simulink model "boostconv"  (R2024a)
settings: Solver=VariableStepAuto  StartTime=0.0  StopTime=10.0  RelTol=1e-3
undefined symbols (not defined in the file): c, l, r, vin
libraries: simulink x1
settings Model: Creator=RAMANJANEYULU  LastModifiedBy=RAMANJANEYULU

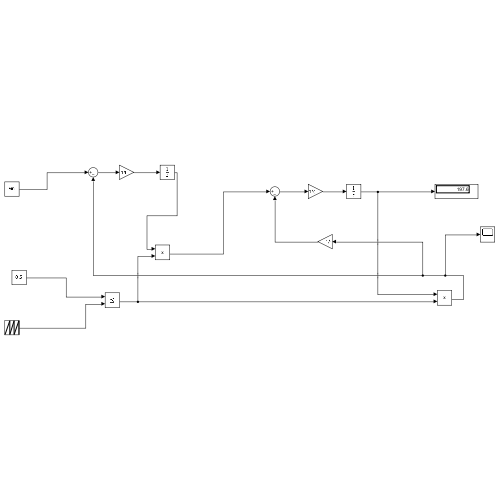
[thumbnail: Simulink's stored preview of the top-level diagram]
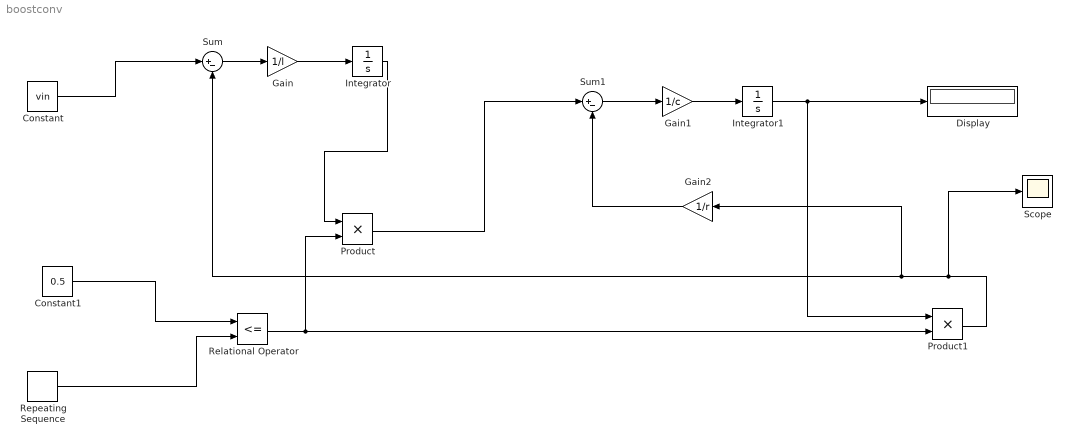
== system boostconv ==
  Constant : Constant  Value=vin
  Constant1 : Constant  Value=0.5
  Display : Display
  Gain : Gain  Gain=1/l
  Gain1 : Gain  Gain=1/c
  Gain2 : Gain  Gain=1/r
  Integrator : Integrator
  Integrator1 : Integrator
  Product : Product
  Product1 : Product
  Relational Operator : RelationalOperator  Operator=<=  OutDataTypeStr=boolean  RndMeth=Simplest  InputSameDT=off
  Repeating Sequence : simulink/Sources/Repeating Sequence  rep_seq_t=[0 1]*1/20000  rep_seq_y=[0 1]
  Scope : Scope
  Sum : Sum  Inputs=|+-
  Sum1 : Sum  Inputs=|+-
  wires:
  Constant/1 -> Sum/1
  Sum/1 -> Gain/1
  Gain/1 -> Integrator/1
  Sum1/1 -> Gain1/1
  Gain1/1 -> Integrator1/1
  Integrator1/1 -> Product1/1, Display/1
  Constant1/1 -> Relational Operator/1
  Repeating Sequence/1 -> Relational Operator/2
  Relational Operator/1 -> Product/2, Product1/2
  Integrator/1 -> Product/1
  Product/1 -> Sum1/1
  Gain2/1 -> Sum1/2
  Product1/1 -> Scope/1, Gain2/1, Sum/2
